simulink model "CalibrationMotorbike"  (R2019a)
settings: Solver=FixedStepDiscrete  StartTime=0.0  StopTime=inf  FixedStep=0.01  RelTol=1e-3  EnableMultiTasking=on
values from neighbouring files (symbols this model uses):
  maxAngleChange_deg = 10.0    [MOCA_DD.sldd]
  maxLongAccNorm_mg = 600.0    [MOCA_DD.sldd]
  minLongAccNorm_mg = 100.0    [MOCA_DD.sldd]
  minSpeedRSD_kmh = 15.0    [MOCA_DD.sldd]
  samplePeriod_s = 0.01    [MOCA_DD.sldd]
libraries: simulink x6
settings Model: DataDictionary=MOCA_DD.sldd  EnableAccessToBaseWorkspace=off  DataTypeOverride=Off  DataTypeOverrideAppliesTo=Floating-point  MinMaxOverflowLogging=ForceOff  Creator=stj1si  LastModifiedBy=HNA3SI
settings DataIOCC: SaveFormat=Array  SaveOutput=off  SignalLogging=off  SaveTime=off  ReturnWorkspaceOutputs=off
settings OptimizationCC: DefaultParameterBehavior=Inlined  DefaultUnderspecifiedDataType=single  InlineInvariantSignals=on  EnhancedBackFolding=on  CachingGlobalReferences=on  ExpressionDepthLimit=2147483647  NoFixptDivByZeroProtection=on  EfficientFloat2IntCast=on  LifeSpan=1  SimCompilerOptimization=on
settings DebuggingCC: SolverPrmCheckMsg=warning  AllowSymbolicDim=off  StateNameClashWarn=warning  SFUnexpectedBacktrackingDiag=warning  SFNoUnconditionalDefaultTransitionDiag=warning  SFExecutionAtInitializationDiag=none  ArithmeticOperatorsInVariantConditions=warning
settings HardwareCC: ProdBitPerPointer=32  ProdBitPerSizeT=32  ProdBitPerPtrDiffT=32  ProdLargestAtomicInteger=Long  ProdLargestAtomicFloat=Double  ProdEndianess=BigEndian  ProdWordSize=32  ProdHWDeviceType=Freescale->32-bit PowerPC
settings ModelReferenceCC: ModelReferenceNumInstancesAllowed=Single  PropagateSignalLabelsOutOfModel=off
settings SFSimCC: SimUseLocalCustomCode=off  MATLABDynamicMemAlloc=off
settings RTWCC: SystemTargetFile=ert.tlc  GenCodeOnly=on  TemplateMakefile=ert_default_tmf  GenerateReport=on  RTWUseLocalCustomCode=off  IncludeHyperlinkInReport=on  LaunchReport=on  GenerateTraceInfo=on  GenerateTraceReport=on  GenerateTraceReportSl=on  GenerateTraceReportSf=on  GenerateTraceReportEml=on
settings CodeAppCC: IgnoreCustomStorageClasses=off  CustomSymbolStrType=$N$R$M  CustomSymbolStrFcnArg=COCA_rt$I$N$M  CustomSymbolStrBlkIO=COCA_rtb_$N$M  StateflowObjectComments=on  InternalIdentifier=Classic
settings ERTTargetCC: TargetLangStandard=C99 (ISO)  MultiwordLength=2048  GenerateSampleERTMain=on  IncludeMdlTerminateFcn=off  CombineSignalStateStructs=on  SuppressErrorStatus=on  SupportNonFinite=off  SupportComplex=off  CastingMode=Standards  InlinedParameterPlacement=NonHierarchical  ERTSrcFileBannerTemplate=ert_code_template_ebike.cgt  ERTCustomFileTemplate=example_file_process.tlc  ERTFilePackagingFormat=Compact  PreserveExternInFcnDecls=off  SuppressUnreachableDefaultCases=off  EnableSignedLeftShifts=off  EnableSignedRightShifts=off  IndentStyle=Allman  EnableUserReplacementTypes=on
settings ConfigComp: CovEnable=on  CovScope=ReferencedModels  CovIncludeTopModel=off  CovMetricSettings=dw  CovHTMLOptions=-sRT=1 -sVT=0 -aTS=1 -bRG=1 -bTC=1 -hTR=0 -nFC=0 -nFD=1 -scm=1 -bcm=1 -xEv=0 -xEM=0  CovHtmlReporting=on  CovSaveCumulativeToWorkspaceVar=on  CovSaveSingleToWorkspaceVar=on  CovModelRefEnable=all  CovSFcnEnable=off

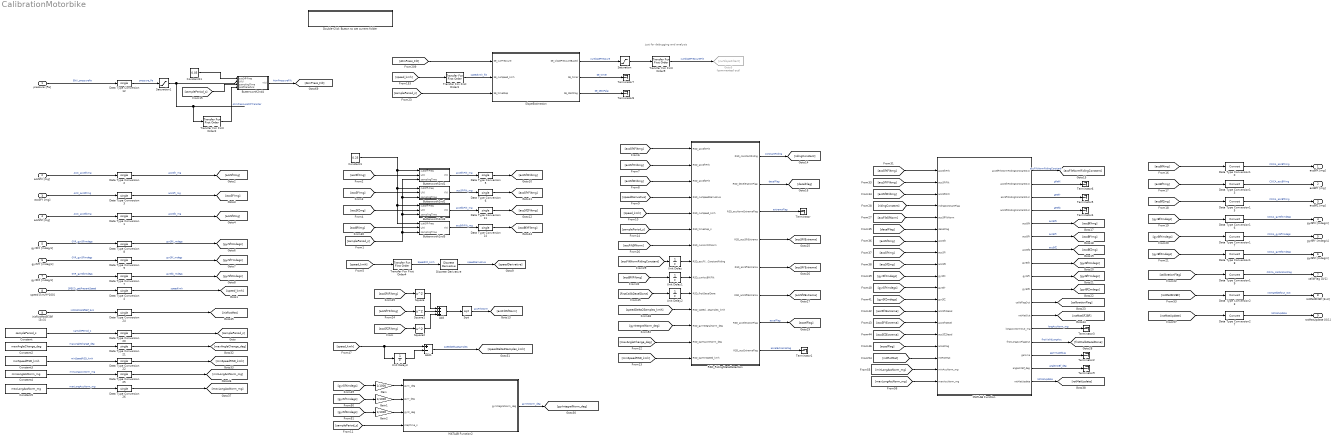
== system CalibrationMotorbike ==
  note: just for debugging and analysis
  "pressure [Pa] " : Inport
  accSfX [mg] : Inport  Port=2
  accSfY [mg] : Inport  Port=3
  accSfZ [mg] : Inport  Port=4
  gyrSfX [mdeg/s] : Inport  Port=5
  gyrSfY [mdeg/s] : Inport  Port=6
  gyrSfZ [mdeg/s] : Inport  Port=7
  speed [km/h*100] : Inport  Port=8
  initRotMatSf2Bf [3x3] : Inport  Port=9  PortDimensions=[3 3]
  Add : Sum  Inputs=+++
  Add1 : Sum  Inputs=+-
  Butterworth2nd1 : Subsystem
  Butterworth2nd2 : Subsystem
  Butterworth2nd3 : Subsystem
  Butterworth2nd4 : Subsystem
  Butterworth2nd5 : Subsystem
  Constant : Constant  Value=samplePeriod_s
  Constant1 : Constant  Value=0.25
  Constant11 : Constant  Value=0.05
  Constant2 : Constant  Value=maxAngleChange_deg
  Constant3 : Constant  Value=minSpeedRSD_kmh
  Constant4 : Constant  Value=minLongAccNorm_mg
  Constant5 : Constant  Value=maxLongAccNorm_mg
  Data Type Conversion{1..9,11..12,14,20..22,24..26} (18 alike) : DataTypeConversion  OutDataTypeStr=single
  Data Type Conversion{10,13,15..19,23,27} (9 alike) : DataTypeConversion  RndMeth=Zero
  Discrete Derivative : simulink/Discrete/Discrete Derivative  gainval=1.0  ICPrevScaledInput=0.0  OutMin=[]  OutMax=[]  OutDataType=fixdt(1, 16)  OutScaling=2^-10  DoSatur=off
  Double-Click Button to set current folder : Subsystem
      settings: OpenFcn=cd(fileparts(get_param(gcs,'filename')));
      mask Display: disp('\bf\fontsize{16}Double-Click to set current folder      ','texmode','on')
  Gain : Gain  Gain=1/1000
  Gain1 : Gain  Gain=1/1000
  Gain2 : Gain  Gain=1/1000
  Goto5 : Goto  Commented=on  GotoTag=curSlopeFilter2
  MATLAB Function : MATLAB Function  TreatAsAtomicUnit=on
  MATLAB Function2 : MATLAB Function  TreatAsAtomicUnit=on
  RSD_RidingStateDetection : Stateflow chart  BlockKeywords=__PRM__SERIALIZED__DATA__:Stateflow Chart,Stateflow Diagram  TreatAsAtomicUnit=on
  Saturation : Saturate  UpperLimit=20  LowerLimit=-20
  Saturation1 : Saturate  UpperLimit=120000  LowerLimit=80000
  SlopeEstimation : Stateflow chart  TreatAsAtomicUnit=on
  Sqrt : Sqrt  SaturateOnIntegerOverflow=on
  Square : Math  Operator=square  SaturateOnIntegerOverflow=on
  Square1 : Math  Operator=square  SaturateOnIntegerOverflow=on
  Square2 : Math  Operator=square  SaturateOnIntegerOverflow=on
  Terminator{,1..9} (10 alike) : Terminator
  Transfer Fcn First Order2 : simulink/Discrete/Transfer Fcn First Order  PoleZ=0.95  ICPrevOutput=90000  DoSatur=off
      settings: SourceProductName=Simulink
  Transfer Fcn First Order3 : simulink/Discrete/Transfer Fcn First Order  PoleZ=0.995  ICPrevOutput=0  DoSatur=off
      settings: SourceProductName=Simulink
  Transfer Fcn First Order4 : simulink/Discrete/Transfer Fcn First Order  PoleZ=0.995  ICPrevOutput=0.0  DoSatur=off
      settings: SourceProductName=Simulink
  Transfer Fcn First Order9 : simulink/Discrete/Transfer Fcn First Order  PoleZ=0.99  ICPrevOutput=0.0  DoSatur=off
      settings: SourceProductName=Simulink
  Unit Delay{,1..3} (4 alike) : UnitDelay  SampleTime=-1  HasFrameUpgradeWarning=on
  accBfX [mg] : Outport
  accBfY [mg] : Outport  Port=2
  accBfZ [mg] : Outport  Port=3
  gyrBfX [mdeg/s] : Outport  Port=4
  gyrBfY [mdeg/s] : Outport  Port=5
  gyrBfZ [mdeg/s] : Outport  Port=6
  calibFlag [0/1] : Outport  Port=7
  rotMatSf2Bf [3x3] : Outport  Port=8
  rotMatUpdate [0/1] : Outport  Port=9
  wires:
  accSfY [mg]/1 -> Data Type Conversion3/1  "ACC_accSfYmg"
  accSfX [mg]/1 -> Data Type Conversion2/1  "ACC_accSfXmg"
  "pressure [Pa] "/1 -> Data Type Conversion12/1  "ENV_pressurePa"
  accSfZ [mg]/1 -> Data Type Conversion1/1  "ACC_accSfZmg"
  gyrSfX [mdeg/s]/1 -> Data Type Conversion8/1  "GYR_gyrSfXmdegs"
  gyrSfY [mdeg/s]/1 -> Data Type Conversion9/1  "GYR_gyrSfYmdegs"
  gyrSfZ [mdeg/s]/1 -> Data Type Conversion7/1  "GYR_gyrSfZmdegs"
  Data Type Conversion10/1 -> accBfX [mg]/1  "COCA_accBfXmg"
  Data Type Conversion13/1 -> accBfY [mg]/1  "COCA_accBfYmg"
  Data Type Conversion15/1 -> accBfZ [mg]/1  "COCA_accBfZmg"
  Data Type Conversion16/1 -> gyrBfX [mdeg/s]/1  "COCA_gyrBfXmdegs"
  Data Type Conversion17/1 -> gyrBfY [mdeg/s]/1  "COCA_gyrBfYmdegs"
  Data Type Conversion18/1 -> gyrBfZ [mdeg/s]/1  "COCA_gyrBfZmdegs"
  Data Type Conversion12/1 -> Saturation1/1  "pressure_Pa"
  Data Type Conversion8/1 -> [gyrSfXmdegs]  "gyrSfX_mdegs"
  Data Type Conversion9/1 -> [gyrSfYmdegs]  "gyrSfY_mdegs"
  Data Type Conversion7/1 -> [gyrSfZmdegs]  "gyrSfZ_mdegs"
  Constant11/1 -> Butterworth2nd4/1(cutOff-Freq)
  [samplePeriod_s] -> Butterworth2nd4/3(samplingTime)
  Butterworth2nd4/1(Y(t)) -> [AtmPress_Filt]  "AtmPressureFilt"
  [samplePeriod_s] -> SlopeEstimation/3(SE_timeStep)
  [AtmPress_Filt] -> SlopeEstimation/1(SE_curPressure)
  SlopeEstimation/1(SE_slopePressureBased) -> Saturation/1  "curSlopePressure"
  [speed_kmh] -> Transfer Fcn First Order3/1
  speed [km/h*100]/1 -> Data Type Conversion4/1  "SPECO_getPresentSpeed"
  [accBfXmg] -> Data Type Conversion10/1
  [accBfYmg] -> Data Type Conversion13/1
  [accBfZmg] -> Data Type Conversion15/1
  [gyrBfXmdegs] -> Data Type Conversion16/1
  [gyrBfYmdegs] -> Data Type Conversion17/1
  [gyrBfZmdegs] -> Data Type Conversion18/1
  Transfer Fcn First Order9/1 -> Goto5/1  "curSlopePressureFilt"
  Transfer Fcn First Order2/1 -> Butterworth2nd4/4(prefilteredVal)  "AtmPressureFiltTransFer"
  Data Type Conversion19/1 -> calibFlag [0/1]/1  "COCA_calibrationFlag"
  [calibrationFlag] -> Data Type Conversion19/1
  Saturation1/1 -> Butterworth2nd4/2(U(t)), Transfer Fcn First Order2/1
  Data Type Conversion4/1 -> [speed_kmh]  "speedKmh"
  Saturation/1 -> Transfer Fcn First Order9/1
  Transfer Fcn First Order3/1 -> SlopeEstimation/2(SE_curSpeed_kmh)  "speedKmh_filt"
  SlopeEstimation/2(SE_timer) -> Terminator7/1  "SE_timer"
  SlopeEstimation/3(SE_2EstFlag) -> Terminator8/1  "SE_2EstFalg"
  Data Type Conversion2/1 -> [accSfXmg]  "accSfX_mg"
  Data Type Conversion3/1 -> [accSfYmg]  "accSfY_mg"
  Data Type Conversion1/1 -> [accSfZmg]  "accSfZ_mg"
  [accSfXmg] -> Butterworth2nd1/2(U(t))
  [accSfYmg] -> Butterworth2nd2/2(U(t))
  [accSfZmg] -> Butterworth2nd3/2(U(t))
  [samplePeriod_s] -> Butterworth2nd5/3(samplingTime), Butterworth2nd1/3(samplingTime), Butterworth2nd2/3(samplingTime), Butterworth2nd3/3(samplingTime)
  Constant1/1 -> Butterworth2nd5/1(cutOff-Freq), Butterworth2nd3/1(cutOff-Freq), Butterworth2nd2/1(cutOff-Freq), Butterworth2nd1/1(cutOff-Freq)
  Butterworth2nd1/1(Y(t)) -> Data Type Conversion5/1  "accSfXFilt_mg"
  Butterworth2nd2/1(Y(t)) -> Data Type Conversion6/1  "accSfYFilt_mg"
  Butterworth2nd3/1(Y(t)) -> Data Type Conversion11/1  "accSfZFilt_mg"
  [speed_kmh] -> Transfer Fcn First Order4/1
  Transfer Fcn First Order4/1 -> Discrete Derivative/1  "SpeedFilt_kmh"
  Discrete Derivative/1 -> [speedDerivative]  "speedDerivative"
  [accSfXFiltmg] -> RSD_RidingStateDetection/1(RSD_accSfXFilt)
  [accSfYFiltmg] -> RSD_RidingStateDetection/2(RSD_accSfYFilt)
  [accSfZFiltmg] -> RSD_RidingStateDetection/3(RSD_accSfZFilt)
  [speedDerivative] -> RSD_RidingStateDetection/4(RSD_curSpeedDerivative)
  [speed_kmh] -> RSD_RidingStateDetection/5(RSD_curSpeed_kmh)
  RSD_RidingStateDetection/1(RSD_constantRiding) -> [ridingConstant]  "constantRiding"
  Data Type Conversion5/1 -> [accSfXFiltmg]
  Data Type Conversion6/1 -> [accSfYFiltmg]
  Data Type Conversion11/1 -> [accSfZFiltmg]
  [samplePeriod_s] -> RSD_RidingStateDetection/6(RSD_timestep_s)
  [accSfXFiltmg] -> Square/1
  [accSfYFiltmg] -> Square1/1
  [accSfZFiltmg] -> Square2/1
  Square1/1 -> Add/2
  Square/1 -> Add/1
  Square2/1 -> Add/3
  Add/1 -> Sqrt/1
  Sqrt/1 -> [accFiltSfNorm]  "accFiltNorm"
  RSD_RidingStateDetection/2(RSD_decelerationFlag) -> [decelFlag]  "decelFlag"
  [accFiltSfNorm] -> MATLAB Function/5(accSfFiltNorm)
  [ridingConstant] -> MATLAB Function/4(ridingConstantFlag)
  MATLAB Function/1(accSfFiltNormRidingConstantOut) -> [accFiltNormRidingConstant]  "accFiltNormRidingConstant"
  [accFiltSfNorm] -> RSD_RidingStateDetection/7(RSD_curAccFiltNorm)
  [accFiltNormRidingConstant] -> Unit Delay/1
  Unit Delay/1 -> RSD_RidingStateDetection/8(RSD_accFiltNormConstantRiding)
  RSD_RidingStateDetection/3(RSD_accNormExtremaFlag) -> Terminator/1  "extremaFlag"
  [accSfXFiltmg] -> MATLAB Function/1(accSfXFilt)
  [accSfYFiltmg] -> MATLAB Function/2(accSfYFilt)
  [accSfZFiltmg] -> MATLAB Function/3(accSfZFilt)
  [decelFlag] -> MATLAB Function/6(decelFlag)
  [accSfXmg] -> MATLAB Function/7(accSfX)
  [accSfYmg] -> MATLAB Function/8(accSfY)
  [accSfZmg] -> MATLAB Function/9(accSfZ)
  MATLAB Function/5(accBfX) -> [accBfXmg]  "accBfX"
  MATLAB Function/6(accBfY) -> [accBfYmg]  "accBfY"
  MATLAB Function/7(accBfZ) -> [accBfZmg]  "accBfZ"
  MATLAB Function/2(accSfXRidingConstantOut) -> Terminator6/1  "gRefX"
  MATLAB Function/3(accSfYRidingConstantOut) -> Terminator5/1  "gRefY"
  MATLAB Function/4(accSfZRidingConstantOut) -> Terminator4/1  "gRefZ"
  MATLAB Function/8(gyrBfX) -> [gyrBfXmdegs]
  MATLAB Function/9(gyrBfY) -> [gyrBfYmdegs]
  MATLAB Function/10(gyrBfZ) -> [gyrBfZmdegs]
  [gyrSfXmdegs] -> MATLAB Function/10(gyrSfX)
  [gyrSfYmdegs] -> MATLAB Function/11(gyrSfY)
  [gyrSfZmdegs] -> MATLAB Function/12(gyrSfZ)
  MATLAB Function/11(calibFlagOut) -> [calibrationFlag]
  [accBfXmg] -> Butterworth2nd5/2(U(t))
  Butterworth2nd5/1(Y(t)) -> Data Type Conversion14/1  "accBfXFilt_mg"
  Data Type Conversion14/1 -> [accBfXFiltmg]
  [accBfXFiltmg] -> Unit Delay1/1
  RSD_RidingStateDetection/4(RSD_accSfXExtrema) -> [accSfXExtrema]
  RSD_RidingStateDetection/5(RSD_accSfYExtrema) -> [accSfYExtrema]
  RSD_RidingStateDetection/6(RSD_accSfZExtrema) -> [accSfZExtrema]
  Unit Delay1/1 -> RSD_RidingStateDetection/9(RSD_curAccBfXFilt)
  [accSfXExtrema] -> MATLAB Function/13(accSfXDecel)
  [accSfYExtrema] -> MATLAB Function/14(accSfYDecel)
  [accSfZExtrema] -> MATLAB Function/15(accSfZDecel)
  MATLAB Function/13(longAccNormOut_mg) -> Terminator3/1  "longAccNorm_mg"
  MATLAB Function/14(firstLongAccFlagOut) -> [firstCalibDecelDone]  "firstValidLongAcc"
  [firstCalibDecelDone] -> Unit Delay2/1
  Unit Delay2/1 -> RSD_RidingStateDetection/10(RSD_firstDecelDone)
  MATLAB Function/15(gamma) -> Terminator2/1  "gammaDebug"
  RSD_RidingStateDetection/7(RSD_accelerationFlag) -> [accelFlag]  "accelFlag"
  RSD_RidingStateDetection/8(RSD_accExtremaFlag) -> Terminator1/1  "accelExtremaFlag"
  [accelFlag] -> MATLAB Function/16(accelFlag)
  [speed_kmh] -> Unit Delay3/1, Add1/1
  Unit Delay3/1 -> Add1/2
  Add1/1 -> [speedDelta2Samples_kmh]  "speedDelta2Samples"
  [speedDelta2Samples_kmh] -> RSD_RidingStateDetection/11(RSD_speedDelta2Samples_kmh)
  [gyrSfZmdegs] -> Gain2/1
  [gyrSfYmdegs] -> Gain1/1
  [gyrSfXmdegs] -> Gain/1
  MATLAB Function2/1(gyrIntegralNorm_deg) -> [gyrIntegralNorm_deg]  "gyrIntNorm_deg"
  [gyrIntegralNorm_deg] -> RSD_RidingStateDetection/12(RSD_gyrIntegralNorm_deg)
  Gain/1 -> MATLAB Function2/1(gyrX_deg)
  Gain1/1 -> MATLAB Function2/2(gyrY_deg)
  Gain2/1 -> MATLAB Function2/3(gyrZ_deg)
  [samplePeriod_s] -> MATLAB Function2/4(stepTime_s)
  Constant/1 -> Data Type Conversion20/1  "samplePeriod_s"
  Data Type Conversion20/1 -> [samplePeriod_s]
  Data Type Conversion21/1 -> [maxAngleChange_deg]
  Constant2/1 -> Data Type Conversion21/1  "maxAngleChange_deg"
  [maxAngleChange_deg] -> RSD_RidingStateDetection/13(RSD_parMaxIntNorm_deg)
  Constant3/1 -> Data Type Conversion22/1  "minSpeedRSD_kmh"
  Data Type Conversion22/1 -> [minSpeedRSD_kmh]
  [minSpeedRSD_kmh] -> RSD_RidingStateDetection/14(RSD_parMinSpeed_kmh)
  MATLAB Function/12(rotMatOut) -> [rotMatSF2BF]
  [rotMatSF2BF] -> Data Type Conversion23/1
  Data Type Conversion23/1 -> rotMatSf2Bf [3x3]/1  "rotMatSf2BfOut_3x3"
  Data Type Conversion24/1 -> [initRotMat]
  initRotMatSf2Bf [3x3]/1 -> Data Type Conversion24/1  "initRotMatSf2Bf_3x3"
  [initRotMat] -> MATLAB Function/17(initRotMat)
  [minLongAccNorm_mg] -> MATLAB Function/18(minAccNorm_mg)
  [maxLongAccNorm_mg] -> MATLAB Function/19(maxAccNorm_mg)
  Data Type Conversion25/1 -> [minLongAccNorm_mg]
  Constant4/1 -> Data Type Conversion25/1  "minLongAccNorm_mg"
  Constant5/1 -> Data Type Conversion26/1  "maxLongAccNorm_mg"
  Data Type Conversion26/1 -> [maxLongAccNorm_mg]
  MATLAB Function/16(angleXZBf_deg) -> Terminator9/1  "angleXZBf_deg"
  [rotMatUpdate] -> Data Type Conversion27/1
  Data Type Conversion27/1 -> rotMatUpdate [0/1]/1  "rotMatUpdate"
  MATLAB Function/17(rotMatUpdate) -> [rotMatUpdate]  "rotMatUpdate"

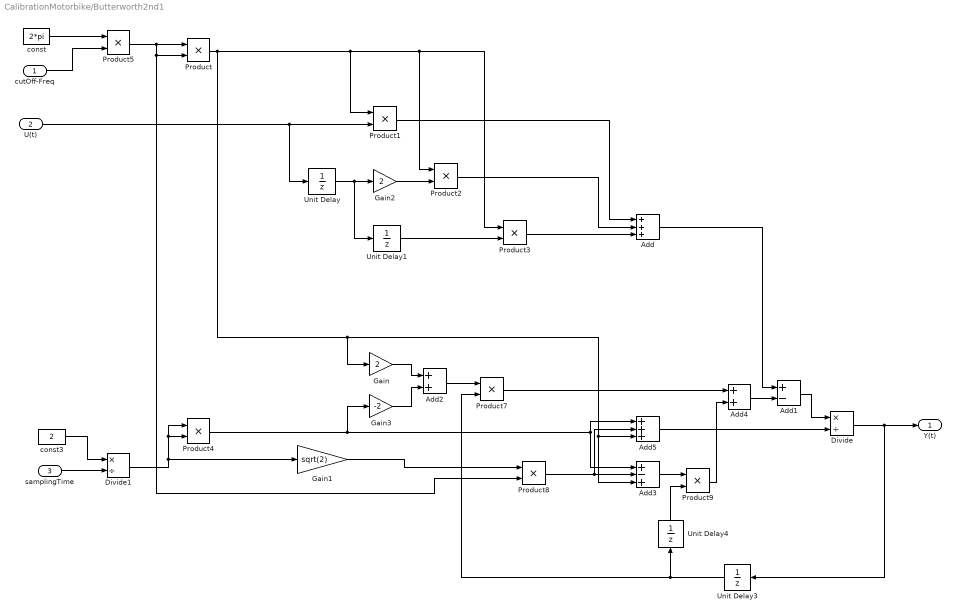
== system CalibrationMotorbike/Butterworth2nd1 ==
  cutOff-Freq : Inport
  U(t) : Inport  Port=2
  samplingTime : Inport  Port=3
  Add : Sum  Inputs=+++
  Add1 : Sum  Inputs=+-
  Add2 : Sum
  Add3 : Sum  Inputs=+-+
  Add4 : Sum
  Add5 : Sum  Inputs=+++
  Divide : Product  Inputs=*/
  Divide1 : Product  Inputs=*/
  Gain : Gain  Gain=2
  Gain1 : Gain  Gain=sqrt(2)
  Gain2 : Gain  Gain=2
  Gain3 : Gain  Gain=-2
  Product{,1..5,7..9} (9 alike) : Product  RndMeth=Zero
  Unit Delay{,1,3..4} (4 alike) : UnitDelay  SampleTime=-1  HasFrameUpgradeWarning=on
  const : Constant  Value=2*pi
  const3 : Constant  Value=2
  Y(t) : Outport
  wires:
  Divide1/1 -> Product4/1, Product4/2, Gain1/1
  samplingTime/1 -> Divide1/2
  const3/1 -> Divide1/1
  cutOff-Freq/1 -> Product5/2
  const/1 -> Product5/1
  Product5/1 -> Product8/2, Product/2, Product/1
  Gain3/1 -> Add2/2
  Gain2/1 -> Product2/2
  Add5/1 -> Divide/2
  Add1/1 -> Divide/1
  Add4/1 -> Add1/2
  Product7/1 -> Add4/1
  Product9/1 -> Add4/2
  Add3/1 -> Product9/1
  Unit Delay4/1 -> Product9/2
  Product8/1 -> Add5/2, Add3/2
  Gain1/1 -> Product8/1
  Add2/1 -> Product7/1
  Unit Delay3/1 -> Unit Delay4/1, Product7/2
  Gain/1 -> Add2/1
  Product4/1 -> Gain3/1, Add5/1, Add3/1
  Divide/1 -> Y(t)/1, Unit Delay3/1
  Add/1 -> Add1/1
  Product3/1 -> Add/3
  Product2/1 -> Add/2
  Product1/1 -> Add/1
  Unit Delay1/1 -> Product3/2
  Unit Delay/1 -> Gain2/1, Unit Delay1/1
  Product/1 -> Add5/3, Add3/3, Gain/1, Product2/1, Product3/1, Product1/1
  U(t)/1 -> Unit Delay/1, Product1/2

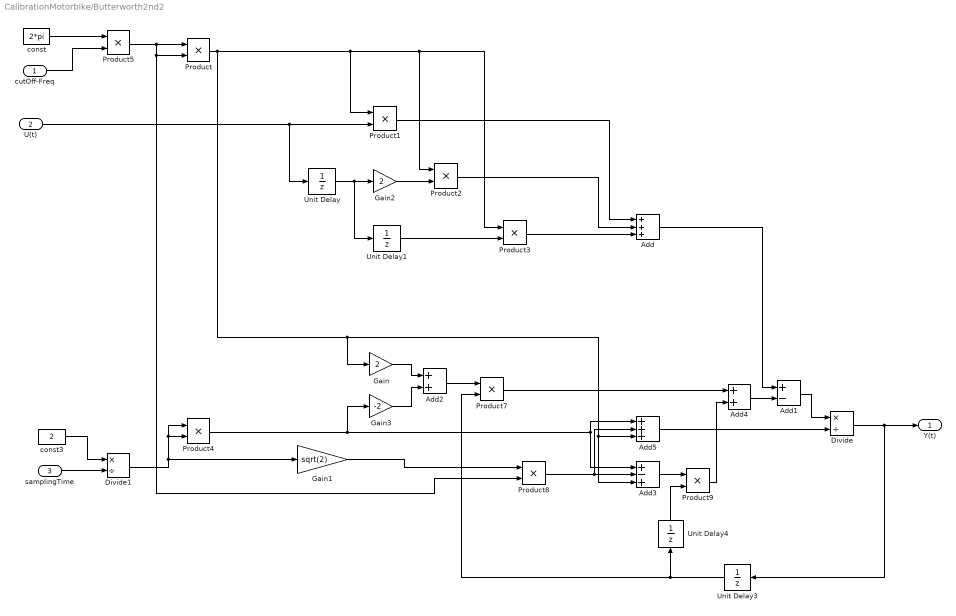
== system CalibrationMotorbike/Butterworth2nd2 ==
  cutOff-Freq : Inport
  U(t) : Inport  Port=2
  samplingTime : Inport  Port=3
  Add : Sum  Inputs=+++
  Add1 : Sum  Inputs=+-
  Add2 : Sum
  Add3 : Sum  Inputs=+-+
  Add4 : Sum
  Add5 : Sum  Inputs=+++
  Divide : Product  Inputs=*/
  Divide1 : Product  Inputs=*/
  Gain : Gain  Gain=2
  Gain1 : Gain  Gain=sqrt(2)
  Gain2 : Gain  Gain=2
  Gain3 : Gain  Gain=-2
  Product{,1..5,7..9} (9 alike) : Product  RndMeth=Zero
  Unit Delay{,1,3..4} (4 alike) : UnitDelay  SampleTime=-1  HasFrameUpgradeWarning=on
  const : Constant  Value=2*pi
  const3 : Constant  Value=2
  Y(t) : Outport
  wires:
  U(t)/1 -> Product1/2, Unit Delay/1
  Product/1 -> Product1/1, Product3/1, Product2/1, Gain/1, Add3/3, Add5/3
  Unit Delay/1 -> Unit Delay1/1, Gain2/1
  Unit Delay1/1 -> Product3/2
  Product1/1 -> Add/1
  Product2/1 -> Add/2
  Product3/1 -> Add/3
  Add/1 -> Add1/1
  Divide/1 -> Unit Delay3/1, Y(t)/1
  Product4/1 -> Add3/1, Add5/1, Gain3/1
  Gain/1 -> Add2/1
  Unit Delay3/1 -> Product7/2, Unit Delay4/1
  Add2/1 -> Product7/1
  Gain1/1 -> Product8/1
  Product8/1 -> Add3/2, Add5/2
  Unit Delay4/1 -> Product9/2
  Add3/1 -> Product9/1
  Product9/1 -> Add4/2
  Product7/1 -> Add4/1
  Add4/1 -> Add1/2
  Add1/1 -> Divide/1
  Add5/1 -> Divide/2
  Gain2/1 -> Product2/2
  Gain3/1 -> Add2/2
  Product5/1 -> Product/1, Product/2, Product8/2
  const/1 -> Product5/1
  cutOff-Freq/1 -> Product5/2
  const3/1 -> Divide1/1
  samplingTime/1 -> Divide1/2
  Divide1/1 -> Gain1/1, Product4/2, Product4/1

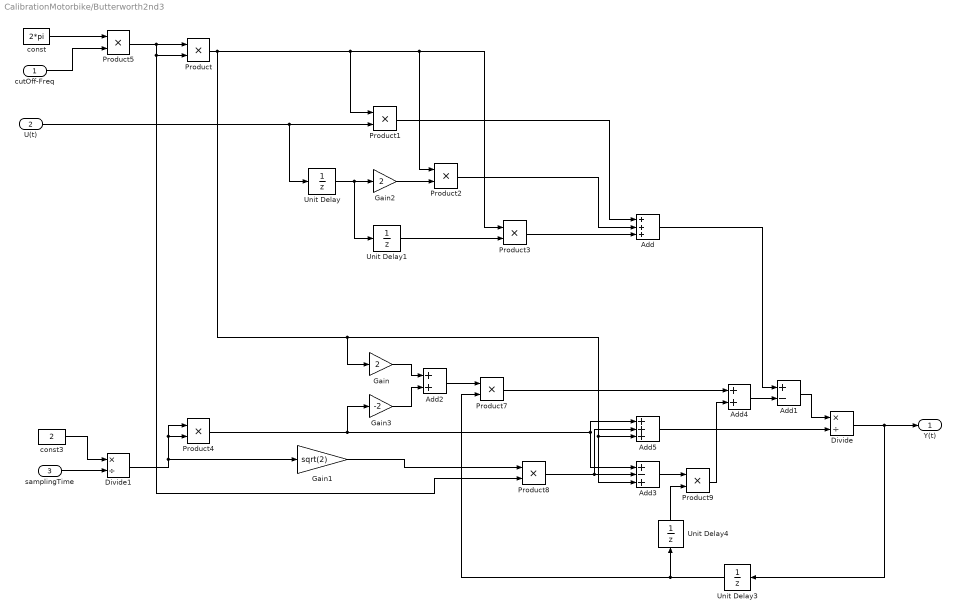
== system CalibrationMotorbike/Butterworth2nd3 ==
  cutOff-Freq : Inport
  U(t) : Inport  Port=2
  samplingTime : Inport  Port=3
  Add : Sum  Inputs=+++
  Add1 : Sum  Inputs=+-
  Add2 : Sum
  Add3 : Sum  Inputs=+-+
  Add4 : Sum
  Add5 : Sum  Inputs=+++
  Divide : Product  Inputs=*/
  Divide1 : Product  Inputs=*/
  Gain : Gain  Gain=2
  Gain1 : Gain  Gain=sqrt(2)
  Gain2 : Gain  Gain=2
  Gain3 : Gain  Gain=-2
  Product{,1..5,7..9} (9 alike) : Product  RndMeth=Zero
  Unit Delay{,1,3..4} (4 alike) : UnitDelay  SampleTime=-1  HasFrameUpgradeWarning=on
  const : Constant  Value=2*pi
  const3 : Constant  Value=2
  Y(t) : Outport
  wires:
  Divide1/1 -> Product4/1, Product4/2, Gain1/1
  samplingTime/1 -> Divide1/2
  const3/1 -> Divide1/1
  cutOff-Freq/1 -> Product5/2
  const/1 -> Product5/1
  Product5/1 -> Product8/2, Product/2, Product/1
  Gain3/1 -> Add2/2
  Gain2/1 -> Product2/2
  Add5/1 -> Divide/2
  Add1/1 -> Divide/1
  Add4/1 -> Add1/2
  Product7/1 -> Add4/1
  Product9/1 -> Add4/2
  Add3/1 -> Product9/1
  Unit Delay4/1 -> Product9/2
  Product8/1 -> Add5/2, Add3/2
  Gain1/1 -> Product8/1
  Add2/1 -> Product7/1
  Unit Delay3/1 -> Unit Delay4/1, Product7/2
  Gain/1 -> Add2/1
  Product4/1 -> Gain3/1, Add5/1, Add3/1
  Divide/1 -> Y(t)/1, Unit Delay3/1
  Add/1 -> Add1/1
  Product3/1 -> Add/3
  Product2/1 -> Add/2
  Product1/1 -> Add/1
  Unit Delay1/1 -> Product3/2
  Unit Delay/1 -> Gain2/1, Unit Delay1/1
  Product/1 -> Add5/3, Add3/3, Gain/1, Product2/1, Product3/1, Product1/1
  U(t)/1 -> Unit Delay/1, Product1/2

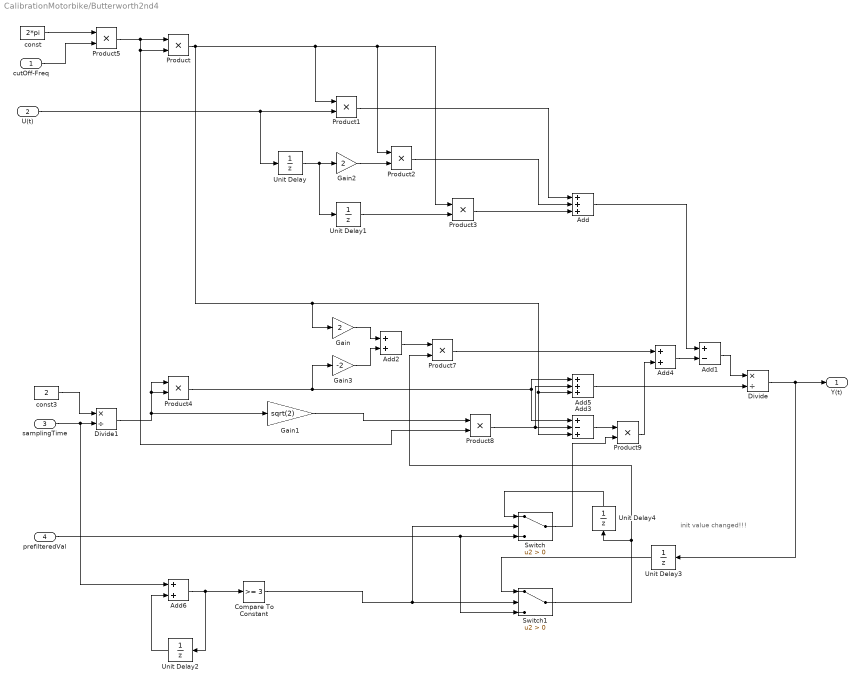
== system CalibrationMotorbike/Butterworth2nd4 ==
  note: init value changed!!!
  cutOff-Freq : Inport
  U(t) : Inport  Port=2
  samplingTime : Inport  Port=3
  prefilteredVal : Inport  Port=4
  Add : Sum  Inputs=+++
  Add1 : Sum  Inputs=+-
  Add2 : Sum
  Add3 : Sum  Inputs=+-+
  Add4 : Sum
  Add5 : Sum  Inputs=+++
  Add6 : Sum
  Compare To Constant : simulink/Logic and Bit Operations/Compare To Constant  relop=>=  const=3  OutDataTypeStr=boolean
  Divide : Product  Inputs=*/
  Divide1 : Product  Inputs=*/
  Gain : Gain  Gain=2
  Gain1 : Gain  Gain=sqrt(2)
  Gain2 : Gain  Gain=2
  Gain3 : Gain  Gain=-2
  Product{,1..5,7..9} (9 alike) : Product  RndMeth=Zero
  Switch : Switch  Criteria=u2 > Threshold
  Switch1 : Switch  Criteria=u2 > Threshold
  Unit Delay{,1..4} (5 alike) : UnitDelay  SampleTime=-1  HasFrameUpgradeWarning=on
  const : Constant  Value=2*pi
  const3 : Constant  Value=2
  Y(t) : Outport
  wires:
  Divide1/1 -> Product4/1, Product4/2, Gain1/1
  samplingTime/1 -> Add6/1, Divide1/2
  const3/1 -> Divide1/1
  cutOff-Freq/1 -> Product5/2
  const/1 -> Product5/1
  Product5/1 -> Product8/2, Product/2, Product/1
  Gain3/1 -> Add2/2
  Gain2/1 -> Product2/2
  Add5/1 -> Divide/2
  Add1/1 -> Divide/1
  Add4/1 -> Add1/2
  Product7/1 -> Add4/1
  Product9/1 -> Add4/2
  Add3/1 -> Product9/1
  Unit Delay4/1 -> Switch/1
  Product8/1 -> Add5/2, Add3/2
  Gain1/1 -> Product8/1
  Add2/1 -> Product7/1
  Gain/1 -> Add2/1
  Product4/1 -> Gain3/1, Add5/1, Add3/1
  Divide/1 -> Y(t)/1, Unit Delay3/1
  Add/1 -> Add1/1
  Product3/1 -> Add/3
  Product2/1 -> Add/2
  Product1/1 -> Add/1
  Unit Delay1/1 -> Product3/2
  Unit Delay/1 -> Gain2/1, Unit Delay1/1
  Product/1 -> Add5/3, Add3/3, Gain/1, Product2/1, Product3/1, Product1/1
  U(t)/1 -> Unit Delay/1, Product1/2
  prefilteredVal/1 -> Switch1/3, Switch/3
  Switch/1 -> Product9/2
  Unit Delay3/1 -> Switch1/1
  Switch1/1 -> Unit Delay4/1, Product7/2
  Add6/1 -> Compare To Constant/1, Unit Delay2/1
  Unit Delay2/1 -> Add6/2
  Compare To Constant/1 -> Switch/2, Switch1/2

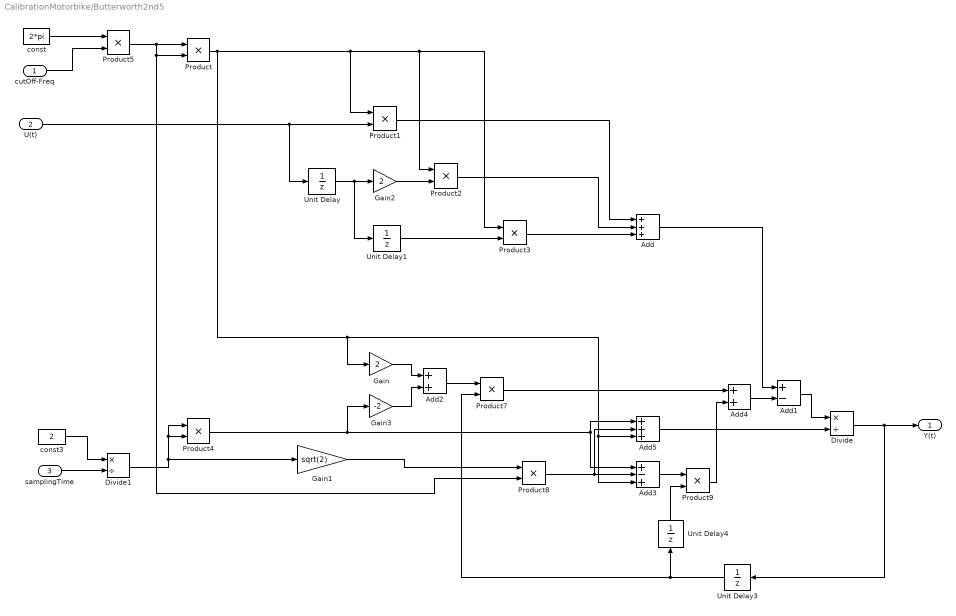
== system CalibrationMotorbike/Butterworth2nd5 ==
  cutOff-Freq : Inport
  U(t) : Inport  Port=2
  samplingTime : Inport  Port=3
  Add : Sum  Inputs=+++
  Add1 : Sum  Inputs=+-
  Add2 : Sum
  Add3 : Sum  Inputs=+-+
  Add4 : Sum
  Add5 : Sum  Inputs=+++
  Divide : Product  Inputs=*/
  Divide1 : Product  Inputs=*/
  Gain : Gain  Gain=2
  Gain1 : Gain  Gain=sqrt(2)
  Gain2 : Gain  Gain=2
  Gain3 : Gain  Gain=-2
  Product{,1..5,7..9} (9 alike) : Product  RndMeth=Zero
  Unit Delay{,1,3..4} (4 alike) : UnitDelay  SampleTime=-1  HasFrameUpgradeWarning=on
  const : Constant  Value=2*pi
  const3 : Constant  Value=2
  Y(t) : Outport
  wires:
  U(t)/1 -> Product1/2, Unit Delay/1
  Product/1 -> Product1/1, Product3/1, Product2/1, Gain/1, Add3/3, Add5/3
  Unit Delay/1 -> Unit Delay1/1, Gain2/1
  Unit Delay1/1 -> Product3/2
  Product1/1 -> Add/1
  Product2/1 -> Add/2
  Product3/1 -> Add/3
  Add/1 -> Add1/1
  Divide/1 -> Unit Delay3/1, Y(t)/1
  Product4/1 -> Add3/1, Add5/1, Gain3/1
  Gain/1 -> Add2/1
  Unit Delay3/1 -> Product7/2, Unit Delay4/1
  Add2/1 -> Product7/1
  Gain1/1 -> Product8/1
  Product8/1 -> Add3/2, Add5/2
  Unit Delay4/1 -> Product9/2
  Add3/1 -> Product9/1
  Product9/1 -> Add4/2
  Product7/1 -> Add4/1
  Add4/1 -> Add1/2
  Add1/1 -> Divide/1
  Add5/1 -> Divide/2
  Gain2/1 -> Product2/2
  Gain3/1 -> Add2/2
  Product5/1 -> Product/1, Product/2, Product8/2
  const/1 -> Product5/1
  cutOff-Freq/1 -> Product5/2
  const3/1 -> Divide1/1
  samplingTime/1 -> Divide1/2
  Divide1/1 -> Gain1/1, Product4/2, Product4/1

== system CalibrationMotorbike/Double-Click Button to set current folder ==

== stateflow chart CalibrationMotorbike/SlopeEstimation ==
  state NotRiding1 [parallel] [commented out]
    en:
  state Riding2 [parallel] [commented out]
    en:
    SE_initPressure = SE_curPressure;
    du:
    SE_deltaAltitude_m = 8434.7 * log(SE_curPressure/SE_initPressure);
    SE_slopePressureBased = atand(SE_deltaAltitude_m/(SE_curSpeed_kmh/3.6*SE_timeStep));
    SE_initPressure = SE_curPressure;
  state Slope1 [parallel]
    settings: executionOrder=1
    state NotRiding
      en:
      SE_2EstFlag = single(0);
    state Riding
      en:
      SE_2EstFlag = single(0);
      SE_initPressure = SE_curPressure;
      SE_curDistanceM = SE_curSpeed_kmh/3.6*SE_timeStep;
    state SpeedIntegration
      en:
      SE_curDistanceM = SE_curSpeed_kmh/3.6*SE_timeStep + SE_curDistanceM;
      SE_timer = SE_timeStep;
      du:
      SE_curDistanceM = SE_curSpeed_kmh/3.6*SE_timeStep + SE_curDistanceM;
      SE_timer = SE_timer + SE_timeStep;
      if SE_timer >= 1
      SE_2EstFlag = single(1);
      end
    state Riding1
      en:
      SE_deltaAltitude_m = 8434.7 * log(SE_curPressure/SE_initPressure);
      SE_asinArg = SE_deltaAltitude_m/SE_curDistanceM;
      if SE_asinArg > 1
      SE_asinArg = single(1);
      elseif SE_asinArg <-1
      SE_asinArg = single(-1);
      end
      SE_slopePressureBased = asind(SE_asinArg);
    (default) -> Slope1.NotRiding : {SE_slopePressureBased = 0;}
    Slope1.SpeedIntegration -> Slope1.NotRiding [order 2] : [SE_curSpeed_kmh < 3]
    Slope1.Riding -> Slope1.NotRiding [order 1] : [SE_curSpeed_kmh < 3]
    Slope1.NotRiding -> Slope1.Riding : [SE_curSpeed_kmh >= 3]
    Slope1.Riding -> Slope1.SpeedIntegration [order 2]
    Slope1.SpeedIntegration -> Slope1.Riding1 [order 1] : [after(2,sec)]
    Slope1.Riding1 -> Slope1.Riding : {
        |
        | }
  state Slope2 [parallel]
    settings: executionOrder=2
    state NotRiding
      en:
    state Riding
      en:
      SE_initPressure2 = SE_curPressure;
      SE_curDistance2M = SE_curSpeed_kmh/3.6*SE_timeStep;
      SE_2EstFlag = single(0);
    state Riding1
      en:
      SE_deltaAltitude_m = 8434.7 * log(SE_curPressure/SE_initPressure2);
      SE_asinArg = SE_deltaAltitude_m/SE_curDistance2M;
      if SE_asinArg > 1
      SE_asinArg = single(1);
      elseif SE_asinArg <-1
      SE_asinArg = single(-1);
      end
      SE_slopePressureBased = asind(SE_asinArg);
    state SpeedIntegration
      en:
      SE_curDistance2M = SE_curSpeed_kmh/3.6*SE_timeStep + SE_curDistance2M;
      du:
      SE_curDistance2M = SE_curSpeed_kmh/3.6*SE_timeStep + SE_curDistance2M;
    (default) -> Slope2.NotRiding : {
        | SE_slopePressureBased = single(0);
        | SE_2EstFlag = single(0);
        | }
    Slope2.Riding1 -> Slope2.NotRiding
    Slope2.SpeedIntegration -> Slope2.NotRiding [order 2] : [SE_curSpeed_kmh < 3]
    Slope2.Riding -> Slope2.NotRiding [order 1] : [SE_curSpeed_kmh < 3]
    Slope2.NotRiding -> Slope2.Riding : [SE_curSpeed_kmh >= 3 && ...
        | SE_2EstFlag == 1]
    Slope2.Riding -> Slope2.SpeedIntegration [order 2]
    Slope2.SpeedIntegration -> Slope2.Riding1 [order 1] : [after(2,sec)]
  (default) -> NotRiding1 [commented out] : {SE_slopePressureBased = 0;}
  Riding2 -> NotRiding1 [commented out] : [SE_curSpeed_kmh < 3]
  NotRiding1 -> Riding2 [commented out] : [SE_curSpeed_kmh >= 3]
  data: SE_curPressure input; SE_curSpeed_kmh input; SE_timeStep input; SE_slopePressureBased output; SE_initPressure local; SE_deltaAltitude_m local; SE_curDistanceM local; SE_curDistance2M local; SE_initPressure2 local; SE_timer output; SE_2EstFlag output; SE_asinArg local

== matlab function CalibrationMotorbike/MATLAB Function ==
  data: accSfXFilt input; accSfFiltNormRidingConstantOut output; accSfYFilt input; accSfZFilt input; ridingConstantFlag input; accSfFiltNorm input; accSfXRidingConstantOut output; accSfYRidingConstantOut output; accSfZRidingConstantOut output; decelFlag input; accSfX input; accSfY input; accSfZ input; accBfX output; accBfY output; accBfZ output; gyrBfX output; gyrBfY output; gyrBfZ output; gyrSfX input; gyrSfY input; gyrSfZ input; calibFlagOut output; rotMatOut output; accSfXDecel input; accSfYDecel input; accSfZDecel input; longAccNormOut_mg output; firstLongAccFlagOut output; gamma output; accelFlag input; initRotMat input; minAccNorm_mg input; maxAccNorm_mg input; angleXZBf_deg output; rotMatUpdate output
function [accSfFiltNormRidingConstantOut, accSfXRidingConstantOut, ...
    accSfYRidingConstantOut, accSfZRidingConstantOut, ...
    accBfX, accBfY, accBfZ, gyrBfX, gyrBfY, gyrBfZ, calibFlagOut, rotMatOut, ...
    longAccNormOut_mg, firstLongAccFlagOut, gamma, angleXZBf_deg, rotMatUpdate]= getDrivingDirection( ...
    accSfXFilt, accSfYFilt, accSfZFilt, ridingConstantFlag, accSfFiltNorm, ...
    decelFlag, accSfX, accSfY, accSfZ, gyrSfX, gyrSfY, gyrSfZ, ...
    accSfXDecel, accSfYDecel, accSfZDecel, accelFlag, initRotMat, ...
    minAccNorm_mg, maxAccNorm_mg)

persistent  accSFFiltNormRidingConstant firstRidindConstantFlag ...
    accSfVecRidingConstant longAccVecSf firstLongAccFlag rotMatSf2Bf calibFlag

if isempty(calibFlag)
    
    if sum(diag(initRotMat)) == 3 || sum(sum(initRotMat))== 0 %not calibrated yet (detect identity matrix or zero matrix)
        rotMatSf2Bf = single(eye(3,3));
        calibFlag = uint16(0);
        firstRidindConstantFlag = uint16(0);
        firstLongAccFlag = uint16(0);
        accSFFiltNormRidingConstant = single(1000);
        accSfVecRidingConstant = single(zeros(3,1));
        longAccVecSf = single(zeros(3,1)); 
    else    %inital calibration is existing
        rotMatSf2Bf = initRotMat;
        calibFlag = uint16(1);
        firstRidindConstantFlag = uint16(1);
        firstLongAccFlag = uint16(2);
        accSFFiltNormRidingConstant = single(1000);
        accSfVecRidingConstant = single(rotMatSf2Bf(3,:)'*1000);
        longAccVecSf = single(rotMatSf2Bf(1,:)');         
    end
end

%when riding constant -> update g-Ref-Vector
if ridingConstantFlag == 1 && firstRidindConstantFlag == 0
    accSFFiltNormRidingConstant = accSfFiltNorm;
    firstRidindConstantFlag = uint16(1);
    accSfVecRidingConstant = [accSfXFilt; accSfYFilt; accSfZFilt;];
elseif ridingConstantFlag == 1 && firstRidindConstantFlag == 1
    accSFFiltNormRidingConstant = 0.9*accSFFiltNormRidingConstant + 0.1*accSfFiltNorm;
    accSfVecRidingConstant = 0.9*accSfVecRidingConstant + 0.1*[accSfXFilt; accSfYFilt; accSfZFilt;];
end

accSfLongAccVec = accSfVecRidingConstant - [accSfXDecel; accSfYDecel; accSfZDecel;];
longAccNorm_mg = norm(accSfLongAccVec);
accSfDecelVecNormed = accSfLongAccVec / longAccNorm_mg;

%when decelerating or accelerating -> update x_BF-Ref-Vector
gamma = single(0);
angleXZBf_deg = single(0);
% if decelFlag == 1 && longAccNorm_mg >= minAccNorm_mg && ...
%         longAccNorm_mg <= maxAccNorm_mg
%     longAccVecSf = accSfDecelVecNormed;
%     %firstLongAccFlag = uint16(1);
% elseif decelFlag == 2 && longAccNorm_mg >= minAccNorm_mg && ...
%         longAccNorm_mg <= maxAccNorm_mg
%     angleXZBf_deg = single(180/pi*atan2(norm(cross(-accSfDecelVecNormed,accSfVecRidingConstant)), dot(-accSfDecelVecNormed,accSfVecRidingConstant)));
%     if abs(angleXZBf_deg - 90) < 12
%         if firstLongAccFlag == 1
%             longAccVecSf = accSfDecelVecNormed; 
%             firstLongAccFlag = uint16(2);
%         else
%             %estimate filter weight
%             gamma = single((longAccNorm_mg - 100)*0.1/150 + 0.05);
%             if gamma > 0.15 %saturation to 15%
%                 gamma = single(0.15);
%             end
%             longAccVecSf = (1-gamma)* longAccVecSf + gamma*accSfDecelVecNormed;
%         end
%     end
% elseif accelFlag == 1 && longAccNorm_mg >= minAccNorm_mg && ...
%         longAccNorm_mg <= maxAccNorm_mg
%     longAccVecSf = -accSfDecelVecNormed;
%     %firstLongAccFlag = uint16(1);
% elseif accelFlag == 2 && longAccNorm_mg >= minAccNorm_mg && ...
%         longAccNorm_mg <= maxAccNorm_mg
%     angleXZBf_deg = single(180/pi*atan2(norm(cross(-accSfDecelVecNormed,accSfVecRidingConstant)), dot(-accSfDecelVecNormed,accSfVecRidingConstant)));
%     if abs(angleXZBf_deg - 90) < 12
%         if firstLongAccFlag == 1
%             longAccVecSf = -accSfDecelVecNormed; 
%             firstLongAccFlag = uint16(2);
%         else
%             %estimate filter weight
%             gamma = single((longAccNorm_mg - 100)*0.1/150 + 0.05);
%             if gamma > 0.15 %saturation to 15%
%                 gamma = single(0.15);
%             end
%             longAccVecSf = (1-gamma)* longAccVecSf - gamma*accSfDecelVecNormed;
%         end
%     end
% end
rotMatUpdate = int16(0);
longAccNormOut_mg = single(0);
%update rotMat only when accelerating of decelerating
if (decelFlag >= 1 || accelFlag >= 1) && longAccNorm_mg >= minAccNorm_mg  &&...
        longAccNorm_mg <= maxAccNorm_mg
    if decelFlag >= 1
        longAccVecSfTmp = accSfDecelVecNormed;
    else
        longAccVecSfTmp = -accSfDecelVecNormed;
    end
    
    %estimate Anlge between longAcc and gRefVector
    angleXZBf_deg = single(180/pi*atan2(norm(...
        cross(-accSfDecelVecNormed,accSfVecRidingConstant)), ...
        dot(-accSfDecelVecNormed,accSfVecRidingConstant)));
    % take only estimates into account, which show of an angle roughly 90° from gRefVector
    
    if firstLongAccFlag == 0 && abs(angleXZBf_deg - 90) < 25 % first longAccEvent with greater angle bandwidth     
        longAccVecSf = longAccVecSfTmp;
        firstLongAccFlag = uint16(1);
        rotMatUpdate = int16(1);
    elseif firstLongAccFlag == 1 && abs(angleXZBf_deg - 90) < 12 
        longAccVecSf = longAccVecSfTmp; 
        firstLongAccFlag = uint16(2);
        calibFlag = uint16(1);
        rotMatUpdate = int16(1);
    elseif firstLongAccFlag == 2 && abs(angleXZBf_deg - 90) < 12 
        %estimate filter weight
        gamma = single((longAccNorm_mg - 100)*0.1/150 + 0.05);
        if gamma > 0.15 %saturation to 15%
            gamma = single(0.15);
        end
        longAccVecSf = (1-gamma)* longAccVecSf + gamma*longAccVecSfTmp;
        rotMatUpdate = int16(1);
    end
    
    
   longAccNormOut_mg = longAccNorm_mg;
   drivingDirectionVec = longAccVecSf;
   accSfRidingConstantVecNormed = accSfVecRidingConstant/norm(accSfVecRidingConstant);
   lateralVec = cross(accSfRidingConstantVecNormed, drivingDirectionVec);
   
   %drivingAxis ->x, lateralAxis ->y, gRefAxis ->z
   rotMatSf2Bf = [drivingDirectionVec';lateralVec'; accSfRidingConstantVecNormed';];
end

% update precision of matrix entries (6 digits after comma) -> finding
% during unitTests (before: different precisions of rotMat in simulation and c!)
rotMatRound = single(fix(rotMatSf2Bf*1e6)*1e-6);

%accBf = rotMatSf2Bf * [accSfX; accSfY; accSfZ;];
%gyrBf = rotMatSf2Bf * [gyrSfX; gyrSfY; gyrSfZ;];
accBf = rotMatRound * [accSfX; accSfY; accSfZ;];
gyrBf = rotMatRound * [gyrSfX; gyrSfY; gyrSfZ;];

accSfXRidingConstantOut = single(accSfVecRidingConstant(1));
accSfYRidingConstantOut = single(accSfVecRidingConstant(2));
accSfZRidingConstantOut = single(accSfVecRidingConstant(3));
accSfFiltNormRidingConstantOut = single(accSFFiltNormRidingConstant);

calibFlagOut = calibFlag;

rotMatOut = single(rotMatRound);

firstLongAccFlagOut = uint16(firstLongAccFlag);

accBfX = single(accBf(1)); 
accBfY = single(accBf(2));
accBfZ = single(accBf(3));

gyrBfX = single(gyrBf(1)); 
gyrBfY = single(gyrBf(2));
gyrBfZ = single(gyrBf(3));

end

== stateflow chart CalibrationMotorbike/RSD_RidingStateDetection ==
  state CheckForConstantRiding [parallel]
    settings: executionOrder=1
    state Idle
      en:
      RSD_constantRiding = uint16(0);
    state WaitState
      en:
      RSD_constantRiding = uint16(0);
    state RidingConstant
      en:
      RSD_constantRiding = uint16(1);
    (default) -> CheckForConstantRiding.Idle : {
        | RSD_constantRiding = uint16(0);
        | }
    CheckForConstantRiding.Idle -> CheckForConstantRiding.WaitState : [RSD_curSpeed_kmh >= RSD_parMinSpeed_kmh && ...
        | abs(RSD_curSpeedDerivative) < 1.5 && ...
        | RSD_gyrIntegralNorm_deg < RSD_parMaxIntNorm_deg]
    CheckForConstantRiding.WaitState -> CheckForConstantRiding.RidingConstant [order 2] : [after(4,sec)]
    CheckForConstantRiding.RidingConstant -> CheckForConstantRiding.WaitState
    CheckForConstantRiding.WaitState -> CheckForConstantRiding.Idle [order 1] : [RSD_curSpeed_kmh < RSD_parMinSpeed_kmh || ...
        | abs(RSD_curSpeedDerivative) >= 1.5 || ...
        | RSD_gyrIntegralNorm_deg >= RSD_parMaxIntNorm_deg || ...
        | RSD_curAccFiltNorm < 850 || RSD_curAccFiltNorm > 1100]
  state CheckForDeceleration [parallel]
    settings: executionOrder=2
    state waitState1
      en:
      RSD_decelerationFlag = uint16(0);
    state RidingConstant
      en:
      RSD_decelerationFlag = uint16(1);
    state Idle
      en:
      RSD_decelerationFlag = uint16(0);
    state WaitState
      en:
      RSD_decelerationFlag = uint16(0);
    state BadSensorData
    state waitState
    state RidingConstant1
      en:
      RSD_decelerationFlag = uint16(2);
    state CheckForINvalidSpeedJump [commented out]
    (default) -> CheckForDeceleration.Idle : {
        | RSD_decelerationFlag = uint16(0);
        | }
    CheckForDeceleration.RidingConstant -> CheckForDeceleration.waitState1
    CheckForDeceleration.waitState1 -> CheckForDeceleration.Idle : [after(10,sec)]
    CheckForDeceleration.RidingConstant1 -> CheckForDeceleration.waitState1
    CheckForDeceleration.WaitState -> CheckForDeceleration.RidingConstant [order 3] : [RSD_accNormExtremaFlag == 1]
    CheckForDeceleration.Idle -> CheckForDeceleration.WaitState [order 2] : %[RSD_curSpeed_kmh >= RSD_parMinSpeed_kmh && ...
        | %RSD_curSpeedDerivative < -5 && after(10,sec)]
        | [RSD_curSpeedDerivative < -5]
    CheckForDeceleration.Idle -> CheckForDeceleration.BadSensorData [order 1] : %bad sensor data
        | [RSD_curAccFiltNorm < 400 || ...
        | RSD_curAccFiltNorm > 1500]
    CheckForDeceleration.BadSensorData -> CheckForDeceleration.waitState : [after(1,sec) && ...
        | RSD_curAccFiltNorm > 400 && ...
        | RSD_curAccFiltNorm < 1500]
    CheckForDeceleration.waitState -> CheckForDeceleration.Idle : [after(10,sec)]
    CheckForDeceleration.WaitState -> CheckForDeceleration.Idle [order 2] : %[RSD_curSpeed_kmh < RSD_parMinSpeed_kmh || ...
        | %RSD_curSpeedDerivative >= -1 || ...
        | %RSD_gyrIntegralNorm_deg >= RSD_parMaxIntNorm_deg]
        | [RSD_curSpeedDerivative >= -1 || ...
        | RSD_gyrIntegralNorm_deg >= RSD_parMaxIntNorm_deg]
    CheckForDeceleration.WaitState -> CheckForDeceleration.RidingConstant1 [order 1] : [RSD_accNormExtremaFlag == 2]
    CheckForDeceleration.WaitState -> CheckForDeceleration.CheckForINvalidSpeedJump [commented out] : [RSD_speedDelta2Samples_kmh > 22]
        | %[abs(RSD_speedDelta2Samples_kmh) > 22]
    CheckForDeceleration.CheckForINvalidSpeedJump -> CheckForDeceleration.Idle [commented out] : [after(10,sec) && ...
        | abs(RSD_curSpeedDerivative) < 2]
    CheckForDeceleration.Idle -> CheckForDeceleration.CheckForINvalidSpeedJump [commented out] : %[RSD_speedDelta2Samples_kmh > 22]
        | [abs(RSD_speedDelta2Samples_kmh) > 22]
  state CheckForAccNormMax [parallel]
    settings: executionOrder=3
    state waitState
    state Idle
      en:
      RSD_accNormExtremaFlag = uint16(0);
    state waitState2
    state Falling
      en:
    state Rising
      en:
    state waitState1
    state Idle2
      en:
      RSD_accNormExtremaFlag = uint16(0);
      RSD_curExtrema = RSD_curAccBfXFilt;
      du:
    state waitState3
    state Falling1
      en:
    (default) -> CheckForAccNormMax.waitState : {
        | RSD_accNormExtremaFlag = uint16(0);
        | }
    CheckForAccNormMax.waitState -> CheckForAccNormMax.Idle : [RSD_constantRiding == 1]
    waitState2 -> CheckForAccNormMax.Idle
    CheckForAccNormMax.waitState1 -> CheckForAccNormMax.Idle
    CheckForAccNormMax.Idle -> Falling [order 3] : [RSD_curAccFiltNorm < RSD_accFiltNormConstantRiding - 25]
        | {RSD_curExtrema = RSD_curAccFiltNorm;}
    CheckForAccNormMax.Idle -> Rising [order 2] : [RSD_curAccFiltNorm > RSD_accFiltNormConstantRiding + 25]
        | {RSD_curExtrema = RSD_curAccFiltNorm;}
    CheckForAccNormMax.Idle -> (junction 109) [order 1] : [RSD_firstDecelDone >= 1]
    Falling -> waitState2 [order 2] : [RSD_curAccFiltNorm > RSD_curExtrema + 4]
        | {
        | RSD_accNormExtremaFlag = uint16(1);
        | }
    Falling -> (junction 109) [order 3] : [RSD_firstDecelDone >= 1]
    Rising -> (junction 109) [order 3] : [RSD_firstDecelDone >= 1]
    Rising -> CheckForAccNormMax.waitState1 [order 2] : [RSD_curAccFiltNorm < RSD_curExtrema - 4]
        | {
        | RSD_accNormExtremaFlag = uint16(1);
        | }
    (junction 109) -> CheckForAccNormMax.Idle2
    Falling -> Falling [order 1] : [RSD_curAccFiltNorm < RSD_curExtrema]
        | {
        | RSD_curExtrema = RSD_curAccFiltNorm;
        | RSD_accSfXExtrema = RSD_accSfXFilt;
        | RSD_accSfYExtrema = RSD_accSfYFilt;
        | RSD_accSfZExtrema = RSD_accSfZFilt;
        | }
    Rising -> Rising [order 1] : [RSD_curAccFiltNorm > RSD_curExtrema]
        | {
        | RSD_curExtrema = RSD_curAccFiltNorm;
        | RSD_accSfXExtrema = RSD_accSfXFilt;
        | RSD_accSfYExtrema = RSD_accSfYFilt;
        | RSD_accSfZExtrema = RSD_accSfZFilt;
        | }
    CheckForAccNormMax.Idle2 -> CheckForAccNormMax.Falling1 [order 2] : [RSD_curAccBfXFilt < RSD_curExtrema - 35]
    CheckForAccNormMax.Idle2 -> CheckForAccNormMax.Idle2 [order 1] : [RSD_curAccBfXFilt > RSD_curExtrema]
        | {
        | RSD_curExtrema = RSD_curAccBfXFilt;
        | }
    CheckForAccNormMax.waitState3 -> CheckForAccNormMax.Idle2
    CheckForAccNormMax.Falling1 -> CheckForAccNormMax.waitState3 [order 1] : [RSD_curAccBfXFilt > RSD_curExtrema + 15]
        | {
        | RSD_accNormExtremaFlag = uint16(2);
        | }
    CheckForAccNormMax.Falling1 -> CheckForAccNormMax.Falling1 [order 2] : [RSD_curAccBfXFilt < RSD_curExtrema]
        | {
        | RSD_curExtrema = RSD_curAccBfXFilt;
        | RSD_accSfXExtrema = RSD_accSfXFilt;
        | RSD_accSfYExtrema = RSD_accSfYFilt;
        | RSD_accSfZExtrema = RSD_accSfZFilt;
        | }
  state CheckForAccelerationPhase [parallel]
    settings: executionOrder=4
    state waitState1
      en:
      RSD_accelerationFlag = uint16(0);
    state RidingConstant
      en:
      RSD_accelerationFlag = uint16(1);
    state Idle
      en:
      RSD_accelerationFlag = uint16(0);
    state WaitState
      en:
      RSD_accelerationFlag = uint16(0);
    state BadSensorData
    state waitState
    state RidingConstant1
      en:
      RSD_accelerationFlag = uint16(2);
    state CheckForINvalidSpeedJump [commented out]
    (default) -> CheckForAccelerationPhase.Idle : {
        | RSD_accelerationFlag = uint16(0);
        | }
    CheckForAccelerationPhase.waitState1 -> CheckForAccelerationPhase.Idle : [after(10,sec)]
    CheckForAccelerationPhase.RidingConstant -> CheckForAccelerationPhase.waitState1
    CheckForAccelerationPhase.RidingConstant1 -> CheckForAccelerationPhase.waitState1
    CheckForAccelerationPhase.WaitState -> CheckForAccelerationPhase.RidingConstant [order 3] : [RSD_accNormExtremaFlag == 1]
    CheckForAccelerationPhase.Idle -> CheckForAccelerationPhase.WaitState [order 2] : %[RSD_curSpeed_kmh >= RSD_parMinSpeed_kmh && ...
        | %RSD_curSpeedDerivative > 5 && after(10,sec)]
        | [RSD_curSpeedDerivative > 5]
    CheckForAccelerationPhase.Idle -> CheckForAccelerationPhase.BadSensorData [order 1] : %bad sensor data
        | [RSD_curAccFiltNorm < 400 || ...
        | RSD_curAccFiltNorm > 1500]
    CheckForAccelerationPhase.waitState -> CheckForAccelerationPhase.Idle : [after(10,sec)]
    CheckForAccelerationPhase.BadSensorData -> CheckForAccelerationPhase.waitState : [after(1,sec) && ...
        | RSD_curAccFiltNorm > 400 && ...
        | RSD_curAccFiltNorm < 1500]
    CheckForAccelerationPhase.WaitState -> CheckForAccelerationPhase.Idle [order 2] : %[RSD_curSpeed_kmh < RSD_parMinSpeed_kmh || ...
        | %RSD_curSpeedDerivative <= 1 || ...
        | %RSD_gyrIntegralNorm_deg >= RSD_parMaxIntNorm_deg]
        | [RSD_curSpeedDerivative <= 1 || ...
        | RSD_gyrIntegralNorm_deg >= RSD_parMaxIntNorm_deg]
    CheckForAccelerationPhase.WaitState -> CheckForAccelerationPhase.RidingConstant1 [order 1] : [RSD_accExtremaFlag == 2]
    CheckForAccelerationPhase.WaitState -> CheckForAccelerationPhase.CheckForINvalidSpeedJump [commented out] : [abs(RSD_speedDelta2Samples_kmh) > 22]
    CheckForAccelerationPhase.CheckForINvalidSpeedJump -> CheckForAccelerationPhase.Idle [commented out] : [after(10,sec) && ...
        | abs(RSD_curSpeedDerivative) < 2]
    CheckForAccelerationPhase.Idle -> CheckForAccelerationPhase.CheckForINvalidSpeedJump [commented out] : [abs(RSD_speedDelta2Samples_kmh) > 22]
  state CheckForAccNormMaxAccelerationPhase [parallel]
    settings: executionOrder=5
    state waitState
    state Idle
      en:
      RSD_accExtremaFlag = uint16(0);
    state Idle2
      en:
      RSD_accExtremaFlag = uint16(0);
      RSD_curAccExtrema = RSD_curAccBfXFilt;
      du:
    state waitState3
    state Falling1
      en:
    (default) -> CheckForAccNormMaxAccelerationPhase.waitState : {
        | RSD_accExtremaFlag = uint16(0);
        | }
    CheckForAccNormMaxAccelerationPhase.waitState -> CheckForAccNormMaxAccelerationPhase.Idle : [RSD_constantRiding == 1]
    CheckForAccNormMaxAccelerationPhase.Idle -> CheckForAccNormMaxAccelerationPhase.Idle2 : [RSD_firstDecelDone >= 1]
    CheckForAccNormMaxAccelerationPhase.Idle2 -> CheckForAccNormMaxAccelerationPhase.Falling1 [order 2] : [RSD_curAccBfXFilt > RSD_curAccExtrema + 35]
    CheckForAccNormMaxAccelerationPhase.Idle2 -> CheckForAccNormMaxAccelerationPhase.Idle2 [order 1] : [RSD_curAccBfXFilt < RSD_curAccExtrema]
        | {
        | RSD_curAccExtrema = RSD_curAccBfXFilt;
        | }
    CheckForAccNormMaxAccelerationPhase.waitState3 -> CheckForAccNormMaxAccelerationPhase.Idle2
    CheckForAccNormMaxAccelerationPhase.Falling1 -> CheckForAccNormMaxAccelerationPhase.waitState3 [order 1] : [RSD_curAccBfXFilt < RSD_curAccExtrema - 15]
        | {
        | RSD_accExtremaFlag = uint16(2);
        | }
    CheckForAccNormMaxAccelerationPhase.Falling1 -> CheckForAccNormMaxAccelerationPhase.Falling1 [order 2] : [RSD_curAccBfXFilt > RSD_curAccExtrema]
        | {
        | RSD_curAccExtrema = RSD_curAccBfXFilt;
        | RSD_accSfXExtrema = RSD_accSfXFilt;
        | RSD_accSfYExtrema = RSD_accSfYFilt;
        | RSD_accSfZExtrema = RSD_accSfZFilt;
        | }
  data: RSD_accSfXFilt input; RSD_accSfYFilt input; RSD_accSfZFilt input; RSD_curSpeedDerivative input; RSD_curSpeed_kmh input; RSD_constantRiding output; RSD_timestep_s input; RSD_gyrYIntegral1 local; RSD_gyrXIntegral1 local; RSD_gyrZIntegral1 local; RSD_decelerationFlag output; RSD_curAccFiltNorm input; RSD_accFiltNormConstantRiding input; RSD_accNormExtremaFlag output; RSD_curExtrema local; RSD_curAccBfXFilt input; RSD_accSfXExtrema output; RSD_accSfYExtrema output; RSD_accSfZExtrema output; RSD_firstDecelDone input uint16; RSD_accelerationFlag output; RSD_curAccExtrema local; RSD_accExtremaFlag output; RSD_speedDelta2Samples_kmh input; RSD_gyrIntegralNorm_deg input; RSD_parMaxIntNorm_deg input; RSD_parMinSpeed_kmh input

== matlab function CalibrationMotorbike/MATLAB Function2 ==
  data: gyrX_deg input; gyrY_deg input; gyrZ_deg input; gyrIntegralNorm_deg output; stepTime_s input
function gyrIntegralNorm_deg  = ...
    orientationChangePastNumSamples(gyrX_deg, gyrY_deg, gyrZ_deg, stepTime_s)

persistent ringBufGyrX ringBufGyrY ringBufGyrZ i
        
numSamples = 300;
%% declaration only during first run!
if isempty(i)  
        ringBufGyrX = single(zeros(numSamples,1));   
        ringBufGyrY = single(zeros(numSamples,1));   
        ringBufGyrZ = single(zeros(numSamples,1));   
        
        i = int16(1); 
end

ringBufGyrX(i) = gyrX_deg;
ringBufGyrY(i) = gyrY_deg;
ringBufGyrZ(i) = gyrZ_deg;

%estimate orientation change in the last 300 samples -> 3s
gyrXIntegral_deg = sum(ringBufGyrX)*stepTime_s;
gyrYIntegral_deg = sum(ringBufGyrY)*stepTime_s;
gyrZIntegral_deg = sum(ringBufGyrZ)*stepTime_s;

gyrIntegralNorm_deg = sqrt(gyrXIntegral_deg^2 + gyrYIntegral_deg^2 + ...
    gyrZIntegral_deg^2);

i = i + 1;
if i > numSamples
    i = int16(1);
end

end
